simulink model "codegen_04"  (R2013b)
settings: Solver=FixedStepDiscrete  StartTime=0.0  StopTime=10.0  FixedStep=0.1  RelTol=1e-3
settings Model: Creator=Administrator  LastModifiedBy=Administrator
settings OptimizationCC: OptimizeModelRefInitCode=on  LifeSpan=1
settings RTWCC: SystemTargetFile=ert.tlc  GenCodeOnly=on  TemplateMakefile=ert_default_tmf  Description=Embedded Coder  GenerateReport=on  ProcessScript=ert_make_rtw_hook  IncludeHyperlinkInReport=on  LaunchReport=on
settings CodeAppCC: IgnoreCustomStorageClasses=off
settings ERTTargetCC: CodeReplacementLibrary=ANSI_C  GenerateSampleERTMain=on  ERTCustomFileTemplate=example_file_process.tlc  EnableUserReplacementTypes=on

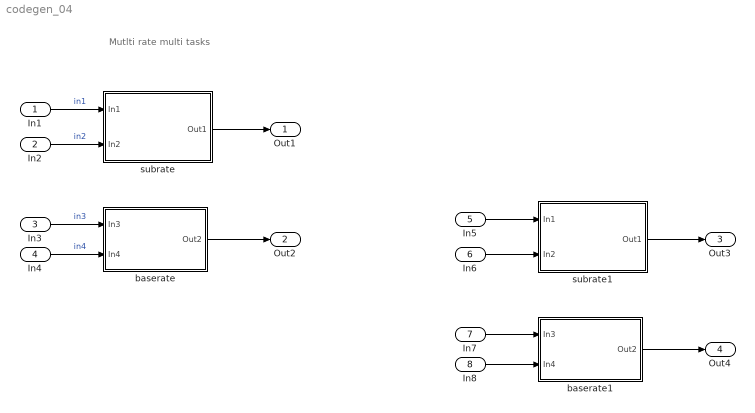
== system codegen_04 ==
  note: Mutlti rate multi tasks
  In1 : Inport  OutDataTypeStr=FLOAT32
  In2 : Inport  Port=2  OutDataTypeStr=UINT16
  In3 : Inport  Port=3  OutDataTypeStr=FLOAT32
  In4 : Inport  Port=4  OutDataTypeStr=UINT16
  In5 : Inport  Port=5  OutDataTypeStr=FLOAT32
  In6 : Inport  Port=6  OutDataTypeStr=UINT16
  In7 : Inport  Port=7  OutDataTypeStr=FLOAT32
  In8 : Inport  Port=8  OutDataTypeStr=UINT16
  baserate : Subsystem  TreatAsAtomicUnit=on
      settings: RTWFcnNameOpts=Use subsystem name
  baserate1 : Subsystem  TreatAsAtomicUnit=on
      settings: RTWFcnNameOpts=Use subsystem name
  subrate : Subsystem  TreatAsAtomicUnit=on  SystemSampleTime=0.6
      settings: RTWFcnNameOpts=Use subsystem name
  subrate1 : Subsystem  TreatAsAtomicUnit=on  SystemSampleTime=0.6
      settings: RTWFcnNameOpts=Use subsystem name
  Out1 : Outport  OutDataTypeStr=boolean
  Out2 : Outport  Port=2  OutDataTypeStr=boolean
  Out3 : Outport  Port=3  OutDataTypeStr=boolean
  Out4 : Outport  Port=4  OutDataTypeStr=boolean
  wires:
  In3/1 -> baserate/1(In3)  "in3"
  In4/1 -> baserate/2(In4)  "in4"
  baserate/1(Out2) -> Out2/1
  In1/1 -> subrate/1(In1)  "in1"
  In2/1 -> subrate/2(In2)  "in2"
  subrate/1(Out1) -> Out1/1
  In7/1 -> baserate1/1(In3)
  In8/1 -> baserate1/2(In4)
  baserate1/1(Out2) -> Out4/1
  In5/1 -> subrate1/1(In1)
  In6/1 -> subrate1/2(In2)
  subrate1/1(Out1) -> Out3/1

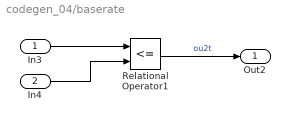
== system codegen_04/baserate ==
  In3 : Inport  OutDataTypeStr=FLOAT32
  In4 : Inport  Port=2  OutDataTypeStr=UINT16
  Relational Operator1 : RelationalOperator  Operator=<=  OutDataTypeStr=boolean
  Out2 : Outport  OutDataTypeStr=boolean
  wires:
  Relational Operator1/1 -> Out2/1  "ou2t"
  In3/1 -> Relational Operator1/1
  In4/1 -> Relational Operator1/2

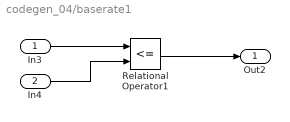
== system codegen_04/baserate1 ==
  In3 : Inport  OutDataTypeStr=FLOAT32
  In4 : Inport  Port=2  OutDataTypeStr=UINT16
  Relational Operator1 : RelationalOperator  Operator=<=  OutDataTypeStr=boolean
  Out2 : Outport  OutDataTypeStr=boolean
  wires:
  Relational Operator1/1 -> Out2/1
  In3/1 -> Relational Operator1/1
  In4/1 -> Relational Operator1/2

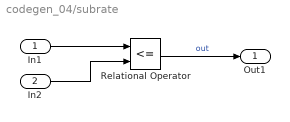
== system codegen_04/subrate ==
  In1 : Inport  OutDataTypeStr=FLOAT32
  In2 : Inport  Port=2  OutDataTypeStr=UINT16
  Relational Operator : RelationalOperator  Operator=<=  OutDataTypeStr=boolean
  Out1 : Outport
  wires:
  In2/1 -> Relational Operator/2
  In1/1 -> Relational Operator/1
  Relational Operator/1 -> Out1/1  "out"

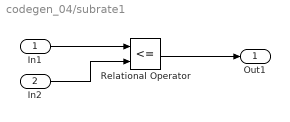
== system codegen_04/subrate1 ==
  In1 : Inport  OutDataTypeStr=FLOAT32
  In2 : Inport  Port=2  OutDataTypeStr=UINT16
  Relational Operator : RelationalOperator  Operator=<=  OutDataTypeStr=boolean
  Out1 : Outport
  wires:
  In2/1 -> Relational Operator/2
  In1/1 -> Relational Operator/1
  Relational Operator/1 -> Out1/1
